simulink model "am"  (R2024b)
settings: Solver=VariableStepAuto  StartTime=0.0  StopTime=10  RelTol=1e-3
libraries: dspfdesign x4, dspvision x4, commchan3 x1
settings Model: Creator=gunes  LastModifiedBy=Asus

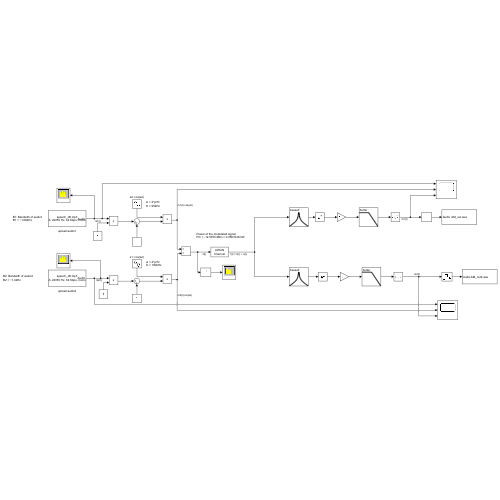
[thumbnail: Simulink's stored preview of the top-level diagram]
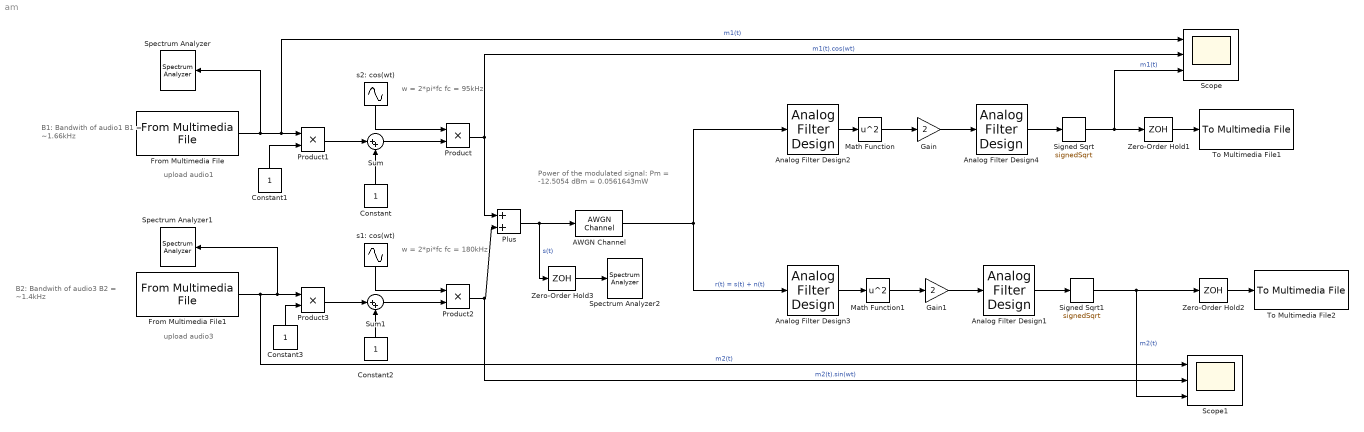
== system am ==
  note: upload audio1
  note: w = 2*pi*fc
      | fc = 95kHz
  note: w = 2*pi*fc
      | fc = 180kHz
  note: B1: Bandwith of audio1
      | B1 = ~1.66kHz
  note: B2: Bandwith of audio3
      | B2 = ~1.4kHz
  note: Power of the modulated signal:
      | Pm = -12.5054 dBm = 0.0561643mW
  note: upload audio3
  AWGN Channel : commchan3/AWGN Channel  LegacyMode=off  NoiseMethod=Variance  noiseMode="Signal to noise ratio  (SNR)"  EbNo=10  EsNo=10  SNR=10  BitsPerSymbol=1  SignalPower=1  SamplesPerSymbol=1  SymbolPeriod=1  VarianceSource=Parameter  Variance=0.0001  RandomStream=Global stream  Seed=67  SimulateUsing=Code generation
  Analog Filter Design1 : dspfdesign/Analog Filter Design  method=Butterworth  filttype=Lowpass  N=8  Wlo=44100  Whi=80  Rp=2  Rs=40
  Analog Filter Design2 : dspfdesign/Analog Filter Design  method=Bessel  filttype=Bandpass  N=8  Wlo=95e3*2*pi  Whi=97e3*2*pi  Rp=2  Rs=40
  Analog Filter Design3 : dspfdesign/Analog Filter Design  method=Bessel  filttype=Bandpass  N=8  Wlo=178e3*2*pi  Whi=2*pi*182e3  Rp=2  Rs=40
  Analog Filter Design4 : dspfdesign/Analog Filter Design  method=Butterworth  filttype=Lowpass  N=8  Wlo=44100  Whi=80  Rp=2  Rs=40
  Constant{,1..3} (4 alike) : Constant
  From Multimedia File : dspvision/From Multimedia File  inputFilename=speech_dft.mp3  readRange=[1 Inf]  loop=on  numPlays=inf  outputStreams=Audio only  videoDataType=single  audioDataType=double  inheritSampleTime=on  userDefinedSampleTime=1/30  noAudioOutput=off  isIntensityVideo=off  fourcc=RGB  colorVideoFormat=Separate color signals  outputEOF=off  dataOrg=Column-major  audioFrameSize=1024  computeAudioFrameSize=off  outSamplingMode=Sample based
      settings: LibrarySourceBlock=audiosources/From Multimedia File
  From Multimedia File1 : dspvision/From Multimedia File  inputFilename=speech_dft.mp3  readRange=[1 Inf]  loop=on  numPlays=inf  outputStreams=Audio only  videoDataType=single  audioDataType=double  inheritSampleTime=on  userDefinedSampleTime=1/30  noAudioOutput=off  isIntensityVideo=off  fourcc=RGB  colorVideoFormat=Separate color signals  outputEOF=off  dataOrg=Column-major  audioFrameSize=1024  computeAudioFrameSize=off  outSamplingMode=Sample based
      settings: LibrarySourceBlock=audiosources/From Multimedia File
  Gain : Gain  Gain=2
  Gain1 : Gain  Gain=2
  Math Function : Math  Operator=square
  Math Function1 : Math  Operator=square
  Plus : Sum
  Product{,1..3} (4 alike) : Product
  Scope : Scope  NumInputPorts=3
  Scope1 : Scope  NumInputPorts=3
  Signed Sqrt : Sqrt  Operator=signedSqrt
  Signed Sqrt1 : Sqrt  Operator=signedSqrt
  Spectrum Analyzer : SpectrumAnalyzer  WindowPosition=[617.000000,142.000000,800.000000,500.000000,]  ScopeFrameLocation=window  WindowInvariantSamplesPerUpdate=on  Span=44100  StartFrequency=-22050  StopFrequency=22050  YLimits=[-106.7236766,-41.56542502]  SelectedToolstripTab=spectrumAnalyzerToolstrip.channelMeasurementsTab
  Spectrum Analyzer1 : SpectrumAnalyzer  WindowPosition=[415.000000,217.000000,800.000000,500.000000,]  ScopeFrameLocation=window  WindowInvariantSamplesPerUpdate=on  Span=44100  StartFrequency=-22050  StopFrequency=22050  YLimits=[-56.27344193,12.7871867]  SelectedToolstripTab=spectrumAnalyzerToolstrip.channelMeasurementsTab
  Spectrum Analyzer2 : SpectrumAnalyzer  WindowPosition=[737.000000,158.000000,800.000000,500.000000,]  ScopeFrameLocation=window  WindowInvariantSamplesPerUpdate=on  Span=44100  StartFrequency=-22050  StopFrequency=22050  YLimits=[-38.35561744,30.73830985]  SelectedToolstripTab=spectrumAnalyzerToolstrip.channelMeasurementsTab
  Sum : Sum  Inputs=|++
  Sum1 : Sum  Inputs=|++
  To Multimedia File1 : dspvision/To Multimedia File  outputFilename=C:\Users\AM_out.wav  streamSelection=Audio only  videoCompressor=None (uncompressed)  audioCompressor=None (uncompressed)  imagePorts=One multidimensional signal  fileType=WAV  audioDatatype=16-bit integer  fourcc=RGB  audioBitRate=128  audioQuality=100  videoQuality=75  mj2000CompFactor=10
      settings: LibrarySourceBlock=dspsnks4/To Multimedia File
  To Multimedia File2 : dspvision/To Multimedia File  outputFilename=C:\Users\AM_out2.wav  streamSelection=Audio only  videoCompressor=None (uncompressed)  audioCompressor=None (uncompressed)  imagePorts=One multidimensional signal  fileType=WAV  audioDatatype=16-bit integer  fourcc=RGB  audioBitRate=128  audioQuality=100  videoQuality=75  mj2000CompFactor=10
      settings: LibrarySourceBlock=dspsnks4/To Multimedia File
  Zero-Order Hold1 : ZeroOrderHold  SampleTime=-1
  Zero-Order Hold2 : ZeroOrderHold  SampleTime=-1
  Zero-Order Hold3 : ZeroOrderHold  SampleTime=-1
  s1: cos(wt) : Sin  Frequency=2*pi*180e3  Phase=-pi/2  SampleTime=0
  s2: cos(wt) : Sin  Frequency=2*pi*95e3  Phase=-pi/2  SampleTime=0
  wires:
  s2: cos(wt)/1 -> Product/1
  Constant/1 -> Sum/2
  Sum/1 -> Product/2
  From Multimedia File/1 -> Product1/1, Scope/1, Spectrum Analyzer/1  "m1(t)"
  Product1/1 -> Sum/1
  Constant1/1 -> Product1/2
  Math Function/1 -> Gain/1
  Gain/1 -> Analog Filter Design4/1
  Analog Filter Design4/1 -> Signed Sqrt/1
  Zero-Order Hold1/1 -> To Multimedia File1/1
  Gain1/1 -> Analog Filter Design1/1
  s1: cos(wt)/1 -> Product2/1
  Constant3/1 -> Product3/2
  Math Function1/1 -> Gain1/1
  From Multimedia File1/1 -> Product3/1, Spectrum Analyzer1/1, Scope1/1  "m2(t)"
  Product2/1 -> Scope1/2, Plus/2  "m2(t).sin(wt)"
  Analog Filter Design1/1 -> Signed Sqrt1/1
  Product3/1 -> Sum1/1
  Constant2/1 -> Sum1/2
  Sum1/1 -> Product2/2
  Signed Sqrt1/1 -> Scope1/3, Zero-Order Hold2/1  "m2(t)"
  Zero-Order Hold2/1 -> To Multimedia File2/1
  Plus/1 -> Zero-Order Hold3/1, AWGN Channel/1  "s(t)"
  Product/1 -> Plus/1, Scope/2  "m1(t).cos(wt)"
  Analog Filter Design2/1 -> Math Function/1
  Analog Filter Design3/1 -> Math Function1/1
  AWGN Channel/1 -> Analog Filter Design3/1, Analog Filter Design2/1  "r(t) = s(t) + n(t)"
  Zero-Order Hold3/1 -> Spectrum Analyzer2/1
  Signed Sqrt/1 -> Scope/3, Zero-Order Hold1/1  "m1(t)"
